simulink model "navigator"  (R2024b)
settings: Solver=FixedStepAuto  StartTime=0.0  StopTime=10.0  FixedStep=0.05  RelTol=1e-3
undefined symbols (not defined in the file or in its folder): CONSTANTS_RADIUS_OF_EARTH, GF_ACTION, GF_MAX_HOR_DIST, GF_MAX_VER_DIST
(part 1 of 2)
settings Model: DataDictionary=nextpilot_datadict.sldd  Creator=DELL  LastModifiedBy=CETCA
settings OptimizationCC: DefaultUnderspecifiedDataType=single
settings DebuggingCC: UnconnectedInputMsg=warning  UnconnectedOutputMsg=warning  UnconnectedLineMsg=warning
settings ModelReferenceCC: EnableRefExpFcnMdlSchedulingChecks=on
settings RTWCC: GPUComputeCapability=3.5  DLArmComputeVersion=19.05

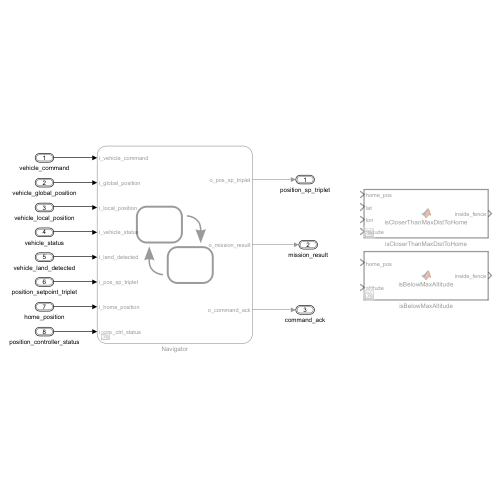
[thumbnail: Simulink's stored preview of the top-level diagram]
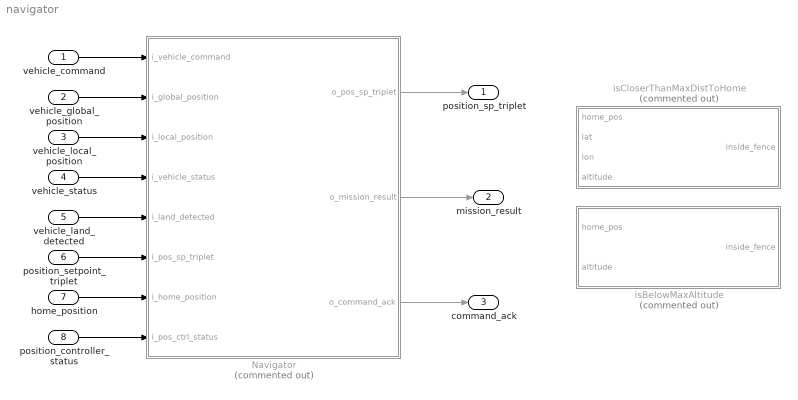
== system navigator ==
  vehicle_command : Inport  OutDataTypeStr=Bus: vehicle_command_s
  vehicle_global_position : Inport  Port=2  OutDataTypeStr=Bus: vehicle_global_position_s
  vehicle_local_position : Inport  Port=3  OutDataTypeStr=Bus: vehicle_local_position_s
  vehicle_status : Inport  Port=4  OutDataTypeStr=Bus: vehicle_status_s
  vehicle_land_detected : Inport  Port=5  OutDataTypeStr=Bus: vehicle_land_detected_s
  position_setpoint_triplet : Inport  Port=6  OutDataTypeStr=Bus: position_setpoint_triplet_s
  home_position : Inport  Port=7  OutDataTypeStr=Bus: home_position_s
  position_controller_status : Inport  Port=8  OutDataTypeStr=Bus: position_controller_status_s
  Navigator : Stateflow chart  Commented=on  TreatAsAtomicUnit=on
  isBelowMaxAltitude : MATLAB Function  Commented=on  TreatAsAtomicUnit=on
  isCloserThanMaxDistToHome : MATLAB Function  Commented=on  TreatAsAtomicUnit=on
  position_sp_triplet : Outport  OutDataTypeStr=Bus: position_setpoint_triplet_s
  mission_result : Outport  Port=2  OutDataTypeStr=Bus: mission_result_s
  command_ack : Outport  Port=3  OutDataTypeStr=Bus: vehicle_command_ack_s
  wires:
  vehicle_command/1 -> Navigator/1(i_vehicle_command)
  vehicle_global_position/1 -> Navigator/2(i_global_position)
  vehicle_local_position/1 -> Navigator/3(i_local_position)
  vehicle_status/1 -> Navigator/4(i_vehicle_status)
  vehicle_land_detected/1 -> Navigator/5(i_land_detected)
  position_setpoint_triplet/1 -> Navigator/6(i_pos_sp_triplet)
  home_position/1 -> Navigator/7(i_home_position)
  position_controller_status/1 -> Navigator/8(i_pos_ctrl_status)
  Navigator/1(o_pos_sp_triplet) -> position_sp_triplet/1
  Navigator/2(o_mission_result) -> mission_result/1
  Navigator/3(o_command_ack) -> command_ack/1

== matlab function navigator/isBelowMaxAltitude ==
  data: home_pos input; inside_fence output; altitude input; GF_MAX_HOR_DIST parameter; GF_MAX_VER_DIST parameter; GF_ACTION parameter
function inside_fence = isBelowMaxAltitude(home_pos,altitude, GF_MAX_HOR_DIST, GF_MAX_VER_DIST, GF_ACTION)

inside_fence = true;

isHomeRequired = (GF_MAX_HOR_DIST > eps) || (GF_MAX_VER_DIST > eps) || (GF_ACTION == GEOFENCE_RESULT.GF_ACTION_RTL);
home_position_valid = (home_pos.timestamp > 0) && home_pos.valid_alt && home_pos.valid_hpos && home_pos.valid_lpos;

if isHomeRequired && home_position_valid
    dist_z = altitude - home_pos.alt;
    
    if (GF_MAX_VER_DIST > eps) && (dist_z > GF_MAX_VER_DIST)
        inside_fence = false;
    end
end

end

== matlab function navigator/isCloserThanMaxDistToHome ==
  data: home_pos input; inside_fence output; lat input; lon input; altitude input; GF_MAX_HOR_DIST parameter; GF_MAX_VER_DIST parameter; GF_ACTION parameter; CONSTANTS_RADIUS_OF_EARTH parameter
function inside_fence = isCloserThanMaxDistToHome(home_pos,lat,lon,altitude, GF_MAX_HOR_DIST, GF_MAX_VER_DIST, GF_ACTION, CONSTANTS_RADIUS_OF_EARTH)

inside_fence = true;

isHomeRequired = (GF_MAX_HOR_DIST > eps) || (GF_MAX_VER_DIST > eps) || (GF_ACTION == GEOFENCE_RESULT.GF_ACTION_RTL);
home_position_valid = (home_pos.timestamp > 0) && home_pos.valid_alt && home_pos.valid_hpos && home_pos.valid_lpos;

if isHomeRequired && home_position_valid
    [dist_xy,~,~] = get_distance_to_point_global_wgs84(lat, lon, altitude, home_pos.lat, home_pos.lon, home_pos.alt, CONSTANTS_RADIUS_OF_EARTH);
    
    if (GF_MAX_HOR_DIST > eps) && (dist_xy > GF_MAX_HOR_DIST)
        inside_fence = false;
    end
end

end
